simulink model "Lee_controller_implementation"  (R2025b)
settings: Solver=FixedStepAuto  StartTime=0.0  StopTime=10  FixedStep=0.001  MaxStep=0.2  RelTol=1e-3
libraries: matrix_library x1
settings Model: Creator=lucag  LastModifiedBy=loren

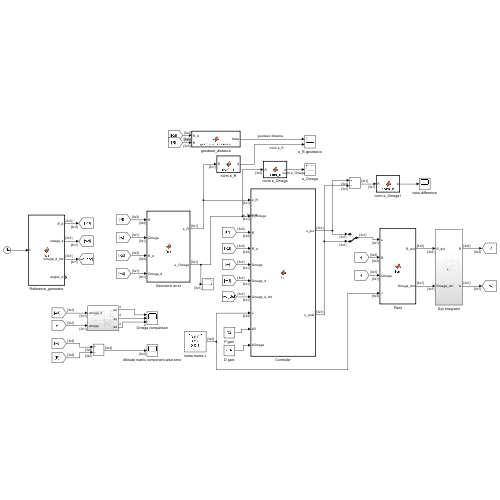
[thumbnail: Simulink's stored preview of the top-level diagram]
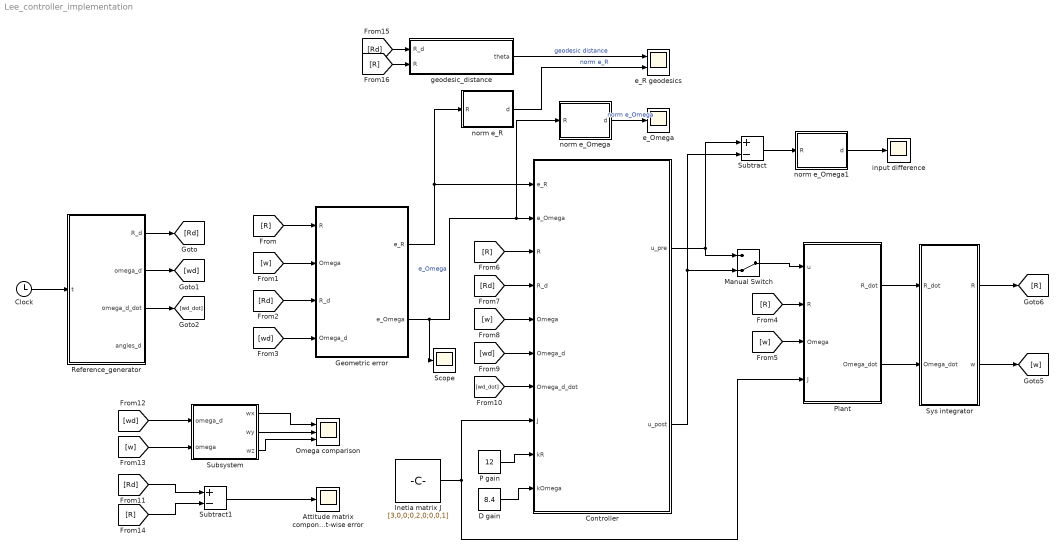
== system Lee_controller_implementation ==
  Attitude matrix component-wise error : Scope
      settings: ActiveDisplayYMinimum=-1  ActiveDisplayYMaximum=1
  Clock : Clock
  Controller : MATLAB Function  TreatAsAtomicUnit=on
  D gain : Constant  Value=8.4
  Geometric error : MATLAB Function  TreatAsAtomicUnit=on
  Inetia matrix J : Constant  Value=[3,0,0;0,2,0;0,0,1]
  Manual Switch : ManualSwitch  CurrentSetting=0
  Omega comparison : Scope  NumInputPorts=3
      settings: ActiveDisplayYMinimum=-10.108397557460609  ActiveDisplayYMaximum=9.1271818153285231  DataLoggingVariableName=ScopeData2
  P gain : Constant  Value=12
  Plant : MATLAB Function  TreatAsAtomicUnit=on
  Reference_generator : MATLAB Function  TreatAsAtomicUnit=on
  Scope : Scope
      settings: ActiveDisplayYMinimum=-1  ActiveDisplayYMaximum=1  DataLoggingVariableName=ScopeData3
  Subsystem : Subsystem
  Subtract : Sum  Inputs=+-
  Subtract1 : Sum  Inputs=+-
  Sys integrator : Subsystem
  e_Omega : Scope
      settings: ActiveDisplayYMinimum=-0.14096284767472422  ActiveDisplayYMaximum=1.4336998957270353  DataLoggingVariableName=ScopeData6
  e_R geodesics : Scope  NumInputPorts=2
      settings: ActiveDisplayYMinimum=-0.39013445320164575  ActiveDisplayYMaximum=3.5336407022420429  DataLoggingVariableName=ScopeData5
  geodesic_distance : MATLAB Function  TreatAsAtomicUnit=on
  input difference : Scope
      settings: ActiveDisplayYMinimum=-0.52939341067580359  ActiveDisplayYMaximum=5.1841004218571776  DataLoggingVariableName=ScopeData4
  norm e_Omega : MATLAB Function  TreatAsAtomicUnit=on
  norm e_Omega1 : MATLAB Function  TreatAsAtomicUnit=on
  norm e_R : MATLAB Function  TreatAsAtomicUnit=on
  wires:
  Clock/1 -> Reference_generator/1(t)
  Controller/1(u_pre) -> Manual Switch/1, Subtract/1
  Reference_generator/1(R_d) -> [Rd]
  Reference_generator/2(omega_d) -> [wd]
  Reference_generator/3(omega_d_dot) -> [wd_dot]
  [w] -> Geometric error/2(Omega)
  [R] -> Geometric error/1(R)
  [Rd] -> Geometric error/3(R_d)
  [wd] -> Geometric error/4(Omega_d)
  [R] -> Controller/3(R)
  [Rd] -> Controller/4(R_d)
  [w] -> Controller/5(Omega)
  [wd] -> Controller/6(Omega_d)
  [wd_dot] -> Controller/7(Omega_d_dot)
  Inetia matrix J/1 -> Plant/4(J), Controller/8(J)
  P gain/1 -> Controller/9(kR)
  D gain/1 -> Controller/10(kOmega)
  [R] -> Plant/2(R)
  [w] -> Plant/3(Omega)
  [wd] -> Subsystem/1(omega_d)
  [w] -> Subsystem/2(omega)
  Subsystem/1(wx) -> Omega comparison/1
  Subsystem/2(wy) -> Omega comparison/2
  Subsystem/3(wz) -> Omega comparison/3
  [Rd] -> Subtract1/1
  [R] -> Subtract1/2
  Subtract1/1 -> Attitude matrix component-wise error/1
  [R] -> geodesic_distance/2(R)
  Geometric error/2(e_Omega) -> Scope/1, norm e_Omega/1(R), Controller/2(e_Omega)  "e_Omega"
  [Rd] -> geodesic_distance/1(R_d)
  Geometric error/1(e_R) -> norm e_R/1(R), Controller/1(e_R)
  norm e_R/1(d) -> e_R geodesics/2  "norm e_R"
  norm e_Omega/1(d) -> e_Omega/1  "norm e_Omega"
  geodesic_distance/1(theta) -> e_R geodesics/1  "geodesic distance"
  Sys integrator/1(R) -> [R]
  Sys integrator/2(w) -> [w]
  Plant/1(R_dot) -> Sys integrator/1(R_dot)
  Plant/2(Omega_dot) -> Sys integrator/2(Omega_dot)
  Controller/2(u_post) -> Manual Switch/2, Subtract/2
  Subtract/1 -> norm e_Omega1/1(R)
  norm e_Omega1/1(d) -> input difference/1
  Manual Switch/1 -> Plant/1(u)

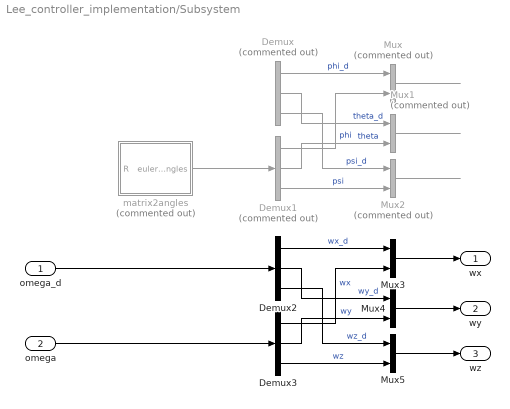
== system Lee_controller_implementation/Subsystem ==
  omega_d : Inport
  omega : Inport  Port=2
  Demux : Demux  Commented=on  Outputs=3
  Demux1 : Demux  Commented=on  Outputs=3
  Demux2 : Demux  Outputs=3
  Demux3 : Demux  Outputs=3
  Mux : Mux  Commented=on  Inputs=2
  Mux1 : Mux  Commented=on  Inputs=2
  Mux2 : Mux  Commented=on  Inputs=2
  Mux3 : Mux  Inputs=2
  Mux4 : Mux  Inputs=2
  Mux5 : Mux  Inputs=2
  matrix2angles : MATLAB Function  Commented=on  TreatAsAtomicUnit=on
  wx : Outport
  wy : Outport  Port=2
  wz : Outport  Port=3
  wires:
  Demux1/2 -> Mux1/2  "theta"
  Demux1/1 -> Mux/2  "phi"
  Demux/1 -> Mux/1  "phi_d"
  ? -> matrix2angles/1(R)
  Demux1/3 -> Mux2/2  "psi"
  matrix2angles/1(euler_angles) -> Demux1/1
  Demux/3 -> Mux2/1  "psi_d"
  ? -> Demux/1
  Demux/2 -> Mux1/1  "theta_d"
  Demux2/2 -> Mux4/1  "wy_d"
  Demux3/2 -> Mux4/2  "wy"
  Demux2/1 -> Mux3/1  "wx_d"
  Demux3/1 -> Mux3/2  "wx"
  Demux3/3 -> Mux5/2  "wz"
  Demux2/3 -> Mux5/1  "wz_d"
  omega/1 -> Demux3/1
  omega_d/1 -> Demux2/1
  Mux/1 -> ?
  Mux1/1 -> ?
  Mux2/1 -> ?
  Mux5/1 -> wz/1
  Mux4/1 -> wy/1
  Mux3/1 -> wx/1

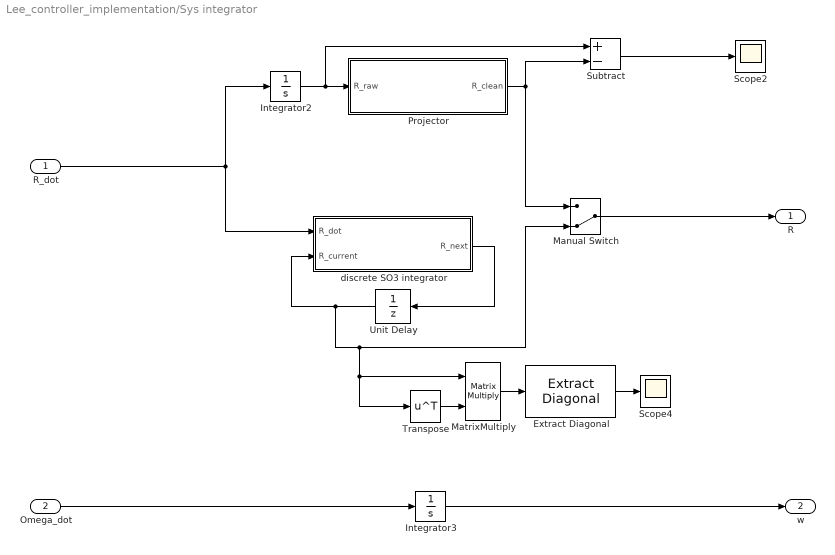
== system Lee_controller_implementation/Sys integrator ==
  R_dot : Inport
  Omega_dot : Inport  Port=2
  Extract Diagonal : matrix_library/Extract Diagonal
      settings: LibrarySourceBlock=|
      | simulink/Matrix
      | Operations/Extract Diagonal
  Integrator2 : Integrator  InitialCondition=eye(3)
  Integrator3 : Integrator  InitialCondition=zeros(3,1)
  Manual Switch : ManualSwitch  CurrentSetting=0
  MatrixMultiply : Product  Multiplication=Matrix(*)
  Projector : MATLAB Function  TreatAsAtomicUnit=on
  Scope2 : Scope
      settings: ActiveDisplayYMinimum=-1  ActiveDisplayYMaximum=1
  Scope4 : Scope
      settings: ActiveDisplayYMinimum=0.99999999999999933  ActiveDisplayYMaximum=1.0000000000000004  DataLoggingVariableName=ScopeData8
  Subtract : Sum  Inputs=+-
  Transpose : Math  Operator=transpose
  Unit Delay : UnitDelay  InitialCondition=eye(3)  SampleTime=1e-3  HasFrameUpgradeWarning=on
  discrete SO3 integrator : MATLAB Function  TreatAsAtomicUnit=on
  R : Outport
  w : Outport  Port=2
  wires:
  discrete SO3 integrator/1(R_next) -> Unit Delay/1
  Extract Diagonal/1 -> Scope4/1
  Subtract/1 -> Scope2/1
  R_dot/1 -> discrete SO3 integrator/1(R_dot), Integrator2/1
  Integrator2/1 -> Subtract/1, Projector/1(R_raw)
  MatrixMultiply/1 -> Extract Diagonal/1
  Unit Delay/1 -> Transpose/1, MatrixMultiply/1, Manual Switch/2, discrete SO3 integrator/2(R_current)
  Projector/1(R_clean) -> Subtract/2, Manual Switch/1
  Transpose/1 -> MatrixMultiply/2
  Integrator3/1 -> w/1
  Omega_dot/1 -> Integrator3/1
  Manual Switch/1 -> R/1

== matlab function Lee_controller_implementation/Sys integrator/Projector ==
  data: R_raw input; R_clean output
function R_clean = fcn(R_raw)
    % This script is used to project back on SO(3) the output of the
    % integrator, which can no longer be a valid rotation matrix due to
    % numerical intgration errors.

    % Perform SVD
    [U, ~, V] = svd(R_raw);
    
    % Reconstruct the closest orthogonal matrix
    R_clean = U * V';
    
    % Ensure determinant is +1 (proper rotation, not reflection)
    if det(R_clean) < 0
        U(:,3) = -U(:,3);
        R_clean = U * V';
    end
end

== matlab function Lee_controller_implementation/Sys integrator/discrete SO3 integrator ==
  data: R_dot input; R_current input; R_next output size=[3 3]
function R_next = discrete_SO3_integrator(R_dot, R_current)

arguments (Input)
    R_dot (3,3)double
    R_current (3,3)double
end
arguments (Output)
    R_next (3,3)double
end
    % discrete_SO3_integrator updates a rotation matrix exactly on the SO(3) manifold.
    % 
    % Inputs:
    %   R_dot     : 3x3 derivative of the rotation matrix
    %   R_current : 3x3 current rotation matrix (feedback from Unit Delay)
    %   dt        : Scalar discrete time step (e.g., 0.01)
    %
    % Output:
    %   R_next    : 3x3 updated rotation matrix for the next time step

    % 1. Extract the skew-symmetric angular velocity matrix [w]x
    % Since R_dot = R * [w]x, we isolate it using [w]x = R^T * R_dot

    dt = 1e-3;
    omega_skew = R_current' * R_dot;
    
    % 2. Extract the angular velocity vector components
    wx = omega_skew(3,2);
    wy = omega_skew(1,3);
    wz = omega_skew(2,1);
    w = [wx; wy; wz];
    
    % 3. Calculate the rotation magnitude
    omega_norm = norm(w);
    theta = omega_norm * dt;
    
    % 4. Compute the Matrix Exponential using Rodrigues' Rotation Formula
    if theta < 1e-7
        % Taylor expansion fallback for very small angles to avoid division by zero
        exp_w_dt = eye(3) + omega_skew * dt;
    else
        % Exact Rodrigues' formula
        u_skew = omega_skew / omega_norm; % Normalized skew matrix
        exp_w_dt = eye(3) + sin(theta) * u_skew + (1 - cos(theta)) * (u_skew * u_skew);
    end
    
    % 5. Apply the discrete update
    R_next = R_current * exp_w_dt;
    
    % 6. Optional but recommended: Numerical stabilization
    % Even though Lie group math is exact, floating-point arithmetic (round-off error) 
    % will slowly degrade orthogonality over millions of time steps. 
    % This first-order projection pulls it strictly back to SO(3).
    R_next = 0.5 * R_next * (3 * eye(3) - R_next' * R_next);
end

== matlab function Lee_controller_implementation/Controller ==
  data: e_R input; e_Omega input; R input; u_pre output; R_d input; Omega input; Omega_d input; Omega_d_dot input; J input; kR input; kOmega input; u_post output
function [u_pre, u_post] = fcn(e_R, e_Omega, R, R_d, Omega, Omega_d, Omega_d_dot, J, kR, kOmega)
    
    % Piece by piece for readability (equation 19, pre-print paper)
    u_fb = -kR * e_R - kOmega * e_Omega;
    u_gyro = cross(Omega, J * Omega);
    term1 = hat(Omega) * R' * R_d * Omega_d;
    term2 = R' * R_d * Omega_d_dot;
    u_ff = -J * (term1 - term2);

    % Total Control
    u_pre = u_fb + u_gyro + u_ff;

    % Piece by piece for readability (equation 23, peer-reviewed paper)
    u_fb = -kR * e_R - kOmega * e_Omega;

    term1 = R' * R_d * Omega_d;
    term2 = J * R' * R_d * Omega_d_dot;
    
    % Total Control
    u_post = u_fb + hat(term1) * J * term1 + term2;
end

function S = hat(v)
    S = [  0,   -v(3),  v(2);
         v(3),   0,    -v(1);
        -v(2),  v(1),   0  ];
end

== matlab function Lee_controller_implementation/Geometric error ==
  data: R input; Omega input; e_R output; R_d input; Omega_d input; e_Omega output
function [e_R, e_Omega] = fcn(R, Omega, R_d, Omega_d)
    % Add max() protection to prevent division-by-zero and complex numbers
    tr_val = max(1 + trace(R_d' * R), eps); 
    
    e_R_matrix = (1 / (2 * sqrt(tr_val))) * (R_d' * R - R' * R_d);
    e_R = vee(e_R_matrix); 
    
    e_Omega = Omega - R' * R_d * Omega_d;
end

function v = vee(S)
    v = [ S(3,2); S(1,3); S(2,1) ];
end

== matlab function Lee_controller_implementation/Plant ==
  data: u input; R input; R_dot output; Omega input; J input; Omega_dot output
function [R_dot, Omega_dot] = fcn(u, R, Omega, J)
    
    % Attitude Kinematics
    R_dot = R * hat(Omega);
    
    % Rigid Body Dynamics
    Omega_dot = J \ (u - cross(Omega, J * Omega));
end

function S = hat(v)
    S = [  0,   -v(3),  v(2);
         v(3),   0,    -v(1);
        -v(2),  v(1),   0  ];
end

== matlab function Lee_controller_implementation/Reference_generator ==
  data: R_d output; omega_d output; omega_d_dot output; angles_d output; t input
function [R_d, omega_d, omega_d_dot, angles_d] = fcn(t)

% Implementation of paper time-dependent reference
phi = 0.999*pi + 0.5*t;
theta = 0.1*t^2;
psi = -0.2*t + 0.5*t^2;

phi_dot = 0.5;
theta_dot = 2*0.1*t;
psi_dot = t-0.2;

phi_ddot = 0;
theta_ddot = 0.2;
psi_ddot = 1;

angles_d = [phi, theta, psi]';

R11 = cos(psi)*cos(theta);
R12 = cos(psi)*sin(theta)*sin(phi) - sin(psi)*cos(phi);
R13 = cos(psi)*sin(theta)*cos(phi) + sin(psi)*sin(phi);
R21 = sin(psi)*cos(theta);
R22 = sin(psi)*sin(theta)*sin(phi) + cos(psi)*cos(phi);
R23 = sin(psi)*sin(theta)*cos(phi) - cos(psi)*sin(phi);
R31 = -sin(theta);
R32 = cos(theta)*sin(phi);
R33 = cos(theta)*cos(phi);

R_d = [R11 R12 R13;
    R21 R22 R23;
    R31 R32 R33];

% 4. Compute Desired Angular Velocity (omega_d)
% Ho dovuto abbandonare la derivazione analitica facendo tutte le derivate
% di tutte le entri della matrice di rotazione altrimenti matlab s
% suicidava. Gemini dice che questo è un modo molt più efficente e
% equivalente. Devo ancora indagare però.
omega_d_1 = phi_dot - psi_dot*sin(theta);
omega_d_2 = theta_dot*cos(phi) + psi_dot*sin(phi)*cos(theta);
omega_d_3 = -theta_dot*sin(phi) + psi_dot*cos(phi)*cos(theta);

omega_d = [omega_d_1, omega_d_2, omega_d_3]';

% Derivative of previous expressions
omega_d_1_dot = phi_ddot - psi_ddot*sin(theta) - psi_dot*theta_dot*cos(theta);

omega_d_2_dot = theta_ddot*cos(phi) - theta_dot*phi_dot*sin(phi) ...
    + psi_ddot*sin(phi)*cos(theta) ...
    + psi_dot*phi_dot*cos(phi)*cos(theta) ...
    - psi_dot*theta_dot*sin(phi)*sin(theta);

omega_d_3_dot = -theta_ddot*sin(phi) - theta_dot*phi_dot*cos(phi) ...
    + psi_ddot*cos(phi)*cos(theta) ...
    - psi_dot*phi_dot*sin(phi)*cos(theta) ...
    - psi_dot*theta_dot*cos(phi)*sin(theta);

omega_d_dot = [omega_d_1_dot, omega_d_2_dot, omega_d_3_dot]';

end

== matlab function Lee_controller_implementation/norm e_Omega1 ==
  data: d output; R input
function d  = norm_e(R)

d = norm(R,2);

end

== matlab function Lee_controller_implementation/Subsystem/matrix2angles ==
  data: euler_angles output; R input
function euler_angles = fcn(R)
    % Extracts 3-2-1 (Yaw-Pitch-Roll) Euler angles from a Rotation Matrix
    % Output: euler_angles = [Roll (phi); Pitch (theta); Yaw (psi)] in radians

    % Extract matrix elements for readability
    r11 = R(1,1);
    r21 = R(2,1);
    r31 = R(3,1);
    r32 = R(3,2);
    r33 = R(3,3);

    % Roll (phi) - rotation about body X axis
    phi = atan2(r32, r33);

    % Pitch (theta) - rotation about body Y axis
    % Note: Using atan2 with the square root instead of asin(-r31) prevents 
    % Simulink from throwing complex number errors due to floating point drift
    theta = atan2(-r31, sqrt(r32^2 + r33^2));

    % Yaw (psi) - rotation about body Z axis
    psi = atan2(r21, r11);

    % Pack into a 3x1 column vector
    euler_angles = [phi; theta; psi];
end

== matlab function Lee_controller_implementation/norm e_R ==
  data: d output; R input
function d  = norm_e(R)

d = norm(R,2);

end

== matlab function Lee_controller_implementation/geodesic_distance ==
  data: theta output; R_d input; R input
function theta  = geodesic_distance(R_d, R)

R = R_d' * R;
theta = acos((trace(R) - 1)/2);
end

== matlab function Lee_controller_implementation/norm e_Omega ==
  data: d output; R input
function d  = norm_e(R)

d = norm(R,2);

end
